simulink model "mobilerobot_DT_SMC"  (R2016b)
settings: Solver=FixedStepAuto  StartTime=0.0  StopTime=20  FixedStep=0.01  RelTol=1e-3
values from neighbouring files (symbols this model uses):
  b = 0.75    [robotprojectvalues.m]
  c = K'    [DTSMC_Gao_TWMR_Position_param.m]    (also in DTSMC_Gao_TWMR_velocity_param.m; robotprojectvalues.m = 0.5)
  c1_pos = c_pos(1)    [robotprojectvalues.m]
  c1_vel = c_vel(1)    [robotprojectvalues.m]
  c2_pos = c_pos(2)    [robotprojectvalues.m]
  c_pos = K_pos'    [robotprojectvalues.m]
  c_vel = K_vel'    [robotprojectvalues.m]
  d = 1    [robotprojectvalues.m]
  dm = 0.1    [robotprojectvalues.m]
  esp = 0.1    [robotprojectvalues.m]
  Gam_tau_pos = [5e-5; 0.01]    [robotprojectvalues.m]
  Gam_tau_vel = [0;1]    [robotprojectvalues.m]
  I_c = 1    [robotprojectvalues.m]
  I_m = 15    [robotprojectvalues.m]
  I_w = 100    [robotprojectvalues.m]
  m1 = a(1)    [robotprojectvalues.m]
  m2 = a(2)    [robotprojectvalues.m]
  m_c = 20    [robotprojectvalues.m]
  m_w = 15    [robotprojectvalues.m]
  mu = 250    [robotprojectvalues.m]
  tau = 0.01    [robotprojectvalues.m]
  x = (1-mu*tau)    (= -1)    [robotprojectvalues.m]
  Xr_c = 5    [robotprojectvalues.m]
  y = dm-esp*tau    (= 0.099)    [robotprojectvalues.m]
  Yr_c = 0    [robotprojectvalues.m]
undefined symbols (not defined in the file or in its folder): fai, Kd, Ki, Kp, theta_dot_L, theta_dot_R
libraries: dspinverses x2, simulink x1
(part 1 of 2)
settings Model: Creator=vasug  LastModifiedBy=HP

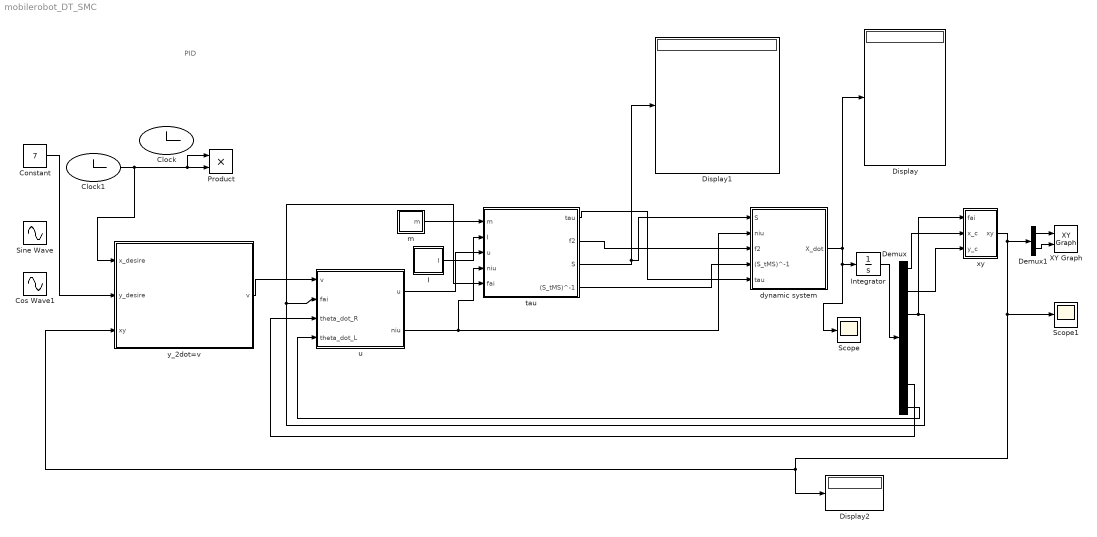
== system mobilerobot_DT_SMC ==
  note: PID
  Clock : Clock
  Clock1 : Clock
  Constant : Constant  Value=7
  Cos Wave1 : Sin  Amplitude=10  Phase=pi/2  SampleTime=0
  Demux : Demux  Outputs=7
  Demux1 : Demux  Outputs=2
  Display : Display
  Display1 : Display
  Display2 : Display
  I : Subsystem
  Integrator : Integrator  InitialCondition=[0; 0; pi/2; 0; 0; 0; 0]
  Product : Product
  Scope : Scope
  Scope1 : Scope
  Sine Wave : Sin  Amplitude=10  SampleTime=0
  XY Graph : simulink/Sinks/XY Graph  xmin=-inf  xmax=inf  ymin=-inf  ymax=inf  st=0.01
  dynamic system : Subsystem
  m : Subsystem
  tau : Subsystem
  "u " : Subsystem
  xy : Subsystem
  y_2dot=v : Subsystem
  wires:
  y_2dot=v/1(v) -> "u "/1(v)
  "u "/1("u ") -> tau/3(u)
  Demux/3 -> xy/1(fai), tau/5(fai), "u "/2(fai)
  tau/4((S_tMS)^-1) -> dynamic system/4((S_tMS)^-1)
  tau/2("f2 ") -> dynamic system/3(f2)
  "u "/2("niu ") -> tau/4(niu), dynamic system/2(niu)
  tau/1(tau) -> dynamic system/5(tau)
  dynamic system/1(X_dot) -> Display/1, Scope/1, Integrator/1
  m/1(m) -> tau/1(m)
  I/1(I) -> tau/2(I)
  xy/1(xy) -> Display2/1, y_2dot=v/3(xy), Scope1/1, Demux1/1
  Demux/1 -> xy/2(x_c)
  Demux/2 -> xy/3(y_c)
  Integrator/1 -> Demux/1
  Demux1/1 -> XY Graph/1
  Demux1/2 -> XY Graph/2
  tau/3("S ") -> Display1/1, dynamic system/1(S)
  Demux/6 -> "u "/3(theta_dot_R)
  Demux/7 -> "u "/4(theta_dot_L)
  Clock1/1 -> y_2dot=v/1(x_desire), Product/1, Product/2
  Constant/1 -> y_2dot=v/2(y_desire)

== system mobilerobot_DT_SMC/I ==
  Constant : Constant  Value=I_c
  Constant1 : Constant  Value=2
  Constant2 : Constant  Value=m_w
  Constant3 : Constant  Value=d
  Constant4 : Constant  Value=b
  Constant5 : Constant  Value=2
  Constant6 : Constant  Value=I_m
  Product : Product
  Product1 : Product  Inputs=3
  Product2 : Product
  Product3 : Product
  Sum : Sum  Inputs=|+++
  Sum1 : Sum  Inputs=|++
  I : Outport
  wires:
  Constant/1 -> Sum/1
  Constant1/1 -> Product1/1
  Constant2/1 -> Product1/2
  Sum1/1 -> Product1/3
  Product1/1 -> Sum/2
  Constant5/1 -> Product/1
  Constant6/1 -> Product/2
  Product/1 -> Sum/3
  Sum/1 -> I/1
  Constant3/1 -> Product2/2, Product2/1
  Product2/1 -> Sum1/1
  Constant4/1 -> Product3/1, Product3/2
  Product3/1 -> Sum1/2

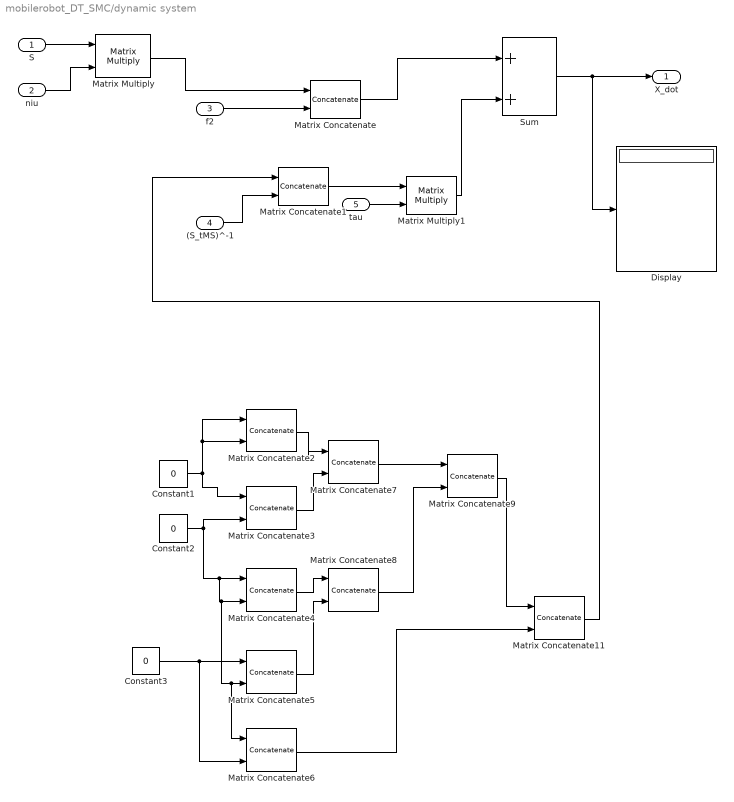
== system mobilerobot_DT_SMC/dynamic system ==
  S : Inport
  niu : Inport  Port=2
  f2 : Inport  Port=3
  (S_tMS)^-1 : Inport  Port=4
  tau : Inport  Port=5
  Constant1 : Constant  Value=0
  Constant2 : Constant  Value=0
  Constant3 : Constant  Value=0
  Display : Display
  Matrix Concatenate{,1,7..9,11} (6 alike) : Concatenate  Mode=Multidimensional array
  Matrix Concatenate{2..6} (5 alike) : Concatenate  Mode=Multidimensional array  ConcatenateDimension=2
  Matrix Multiply : Product  Multiplication=Matrix(*)
  Matrix Multiply1 : Product  Multiplication=Matrix(*)
  Sum : Sum  Inputs=|++
  X_dot : Outport
  wires:
  niu/1 -> Matrix Multiply/2
  S/1 -> Matrix Multiply/1
  Matrix Multiply/1 -> Matrix Concatenate/1
  f2/1 -> Matrix Concatenate/2
  Matrix Concatenate/1 -> Sum/1
  (S_tMS)^-1/1 -> Matrix Concatenate1/2
  Sum/1 -> Display/1, X_dot/1
  Matrix Concatenate1/1 -> Matrix Multiply1/1
  tau/1 -> Matrix Multiply1/2
  Matrix Multiply1/1 -> Sum/2
  Matrix Concatenate6/1 -> Matrix Concatenate11/2
  Matrix Concatenate9/1 -> Matrix Concatenate11/1
  Matrix Concatenate4/1 -> Matrix Concatenate8/1
  Matrix Concatenate5/1 -> Matrix Concatenate8/2
  Matrix Concatenate7/1 -> Matrix Concatenate9/1
  Constant2/1 -> Matrix Concatenate3/2, Matrix Concatenate6/1, Matrix Concatenate5/2, Matrix Concatenate4/2, Matrix Concatenate4/1
  Matrix Concatenate2/1 -> Matrix Concatenate7/1
  Matrix Concatenate3/1 -> Matrix Concatenate7/2
  Matrix Concatenate8/1 -> Matrix Concatenate9/2
  Constant1/1 -> Matrix Concatenate3/1, Matrix Concatenate2/2, Matrix Concatenate2/1
  Matrix Concatenate11/1 -> Matrix Concatenate1/1
  Constant3/1 -> Matrix Concatenate6/2, Matrix Concatenate5/1

== system mobilerobot_DT_SMC/m ==
  Constant : Constant  Value=m_c
  Constant2 : Constant  Value=m_w
  Constant3 : Constant  Value=2
  Product : Product
  Sum : Sum  Inputs=|++
  m : Outport
  wires:
  Constant3/1 -> Product/1
  Constant2/1 -> Product/2
  Product/1 -> Sum/2
  Constant/1 -> Sum/1
  Sum/1 -> m/1

== system mobilerobot_DT_SMC/tau ==
  m : Inport
  I : Inport  Port=2
  u : Inport  Port=3
  niu : Inport  Port=4
  fai : Inport  Port=5
  Derivative : Derivative
  Display : Display
  M : Subsystem
  Matrix Multiply : Product  Inputs=3  Multiplication=Matrix(*)
  Matrix Multiply1 : Product  Multiplication=Matrix(*)
  Product : Product
  S : Subsystem
  "S_transpose " : Subsystem
  Sum : Sum  Inputs=|+-
  f2 : Subsystem
  tau : Outport
  "f2 " : Outport  Port=2
  "S " : Outport  Port=3
  (S_tMS)^-1 : Outport  Port=4
  wires:
  I/1 -> f2/2(I), M/3("I ")
  fai/1 -> Derivative/1, S/1("fai "), f2/3(fai), M/1("fai "), "S_transpose "/1("fai ")
  m/1 -> M/2("m "), f2/1(m)
  "S_transpose "/1(S_t) -> Matrix Multiply/1
  M/1(M) -> Matrix Multiply/2
  S/1(S) -> "S "/1, Matrix Multiply/3
  f2/1(f2) -> Sum/2, "f2 "/1
  u/1 -> Sum/1
  Sum/1 -> Matrix Multiply1/2
  Matrix Multiply/1 -> Matrix Multiply1/1
  Matrix Multiply1/1 -> tau/1
  f2/2((S_tMS)^-1) -> (S_tMS)^-1/1
  Derivative/1 -> Product/2, Product/1
  Product/1 -> Display/1, f2/5((fai_dot)^2)
  niu/1 -> f2/4(niu)

== system mobilerobot_DT_SMC/u  ==
  v : Inport
  fai : Inport  Port=2
  theta_dot_R : Inport  Port=3
  theta_dot_L : Inport  Port=4
  Display4 : Display
  Display8 : Display
  Matrix Multiply : Product  Multiplication=Matrix(*)
  Matrix Multiply1 : Product  Multiplication=Matrix(*)
  Sum : Sum  Inputs=|+-
  faifunction dot : Subsystem
  inverse faifunction : Subsystem
  "niu " : Subsystem
  "u " : Outport
  "niu " : Outport  Port=2
  wires:
  faifunction dot/1(Out1) -> Matrix Multiply/1, Display4/1
  fai/1 -> faifunction dot/1(fai), inverse faifunction/1(fai)
  v/1 -> Sum/1
  inverse faifunction/1(Out1) -> Matrix Multiply1/1, Display8/1
  "niu "/1(Out1) -> Matrix Multiply/2, "niu "/1
  Matrix Multiply/1 -> Sum/2
  Matrix Multiply1/1 -> "u "/1
  Sum/1 -> Matrix Multiply1/2
  theta_dot_L/1 -> "niu "/2(theta_dot_L)
  theta_dot_R/1 -> "niu "/1(theta_dot_R)

== system mobilerobot_DT_SMC/xy ==
  fai : Inport
  x_c : Inport  Port=2
  y_c : Inport  Port=3
  Display : Display
  Matrix Concatenate : Concatenate
  Xr : Subsystem
  Yr : Subsystem
  xy : Outport
  wires:
  Yr/1(Out1) -> Matrix Concatenate/2
  Matrix Concatenate/1 -> Display/1, xy/1
  Xr/1(Out1) -> Matrix Concatenate/1
  fai/1 -> Xr/1(fai), Yr/1("fai ")
  x_c/1 -> Xr/2(Xc)
  y_c/1 -> Yr/2("Yc ")

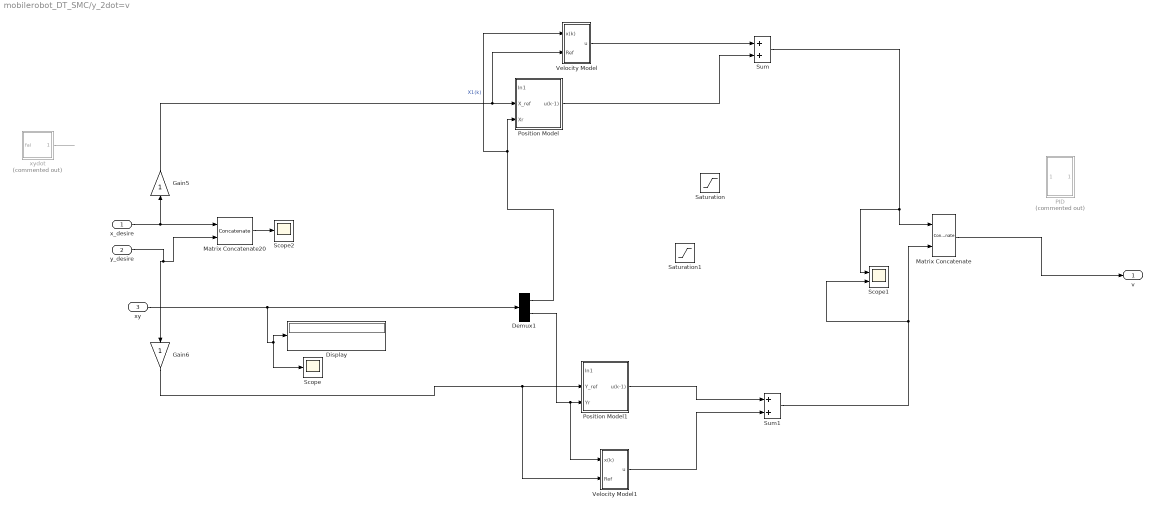
== system mobilerobot_DT_SMC/y_2dot=v ==
  x_desire : Inport
  y_desire : Inport  Port=2
  xy : Inport  Port=3
  Demux1 : Demux  Outputs=2
  Display : Display
  Gain5 : Gain
  Gain6 : Gain
  Matrix Concatenate : Concatenate  Mode=Multidimensional array
  Matrix Concatenate20 : Concatenate  Mode=Multidimensional array
  PID : Subsystem  Commented=on
  Position Model : Subsystem
  Position Model1 : Subsystem
  Saturation : Saturate  UpperLimit=50  LowerLimit=-50  LinearizeAsGain=off
  Saturation1 : Saturate  UpperLimit=50  LowerLimit=-50  LinearizeAsGain=off
  Scope : Scope
  Scope1 : Scope  NumInputPorts=2
  Scope2 : Scope
  Sum : Sum
  Sum1 : Sum
  Velocity Model : Subsystem
  Velocity Model1 : Subsystem
  xydot : Subsystem  Commented=on
  v : Outport
  wires:
  xydot/1(Out1) -> ?
  xy/1 -> Demux1/1, Scope/1, Display/1
  Matrix Concatenate/1 -> v/1
  x_desire/1 -> Matrix Concatenate20/1, Gain5/1
  y_desire/1 -> Matrix Concatenate20/2, Gain6/1
  Matrix Concatenate20/1 -> Scope2/1
  Gain5/1 -> Velocity Model/2(Ref), Position Model/2(X_ref)
  Demux1/1 -> Velocity Model/1(x(k)), Position Model/3(Xr)  "X1(k)"
  Velocity Model/1(u) -> Sum/1
  Position Model/1(u(k-1)) -> Sum/2
  Sum/1 -> Scope1/1, Matrix Concatenate/1
  Gain6/1 -> Velocity Model1/2(Ref), Position Model1/2(Y_ref)
  Demux1/2 -> Velocity Model1/1(x(k)), Position Model1/3(Yr)
  Velocity Model1/1(u) -> Sum1/2
  Position Model1/1(u(k-1)) -> Sum1/1
  Sum1/1 -> Scope1/2, Matrix Concatenate/2

== system mobilerobot_DT_SMC/tau/M ==
  "fai " : Inport
  "m " : Inport  Port=2
  "I " : Inport  Port=3
  Constant : Constant  Value=I_w
  Constant1 : Constant  Value=0
  Constant3 : Constant  Value=0
  Constant5 : Constant  Value=0
  Matrix Concatenate{,1..4} (5 alike) : Concatenate  NumInputs=5  Mode=Multidimensional array  ConcatenateDimension=2
  Matrix Concatenate7 : Concatenate  NumInputs=5  Mode=Multidimensional array
  Subsystem : Subsystem
  Subsystem1 : Subsystem
  M : Outport
  wires:
  "m "/1 -> Matrix Concatenate1/2, Matrix Concatenate/1
  Constant5/1 -> Matrix Concatenate/2
  "fai "/1 -> Subsystem1/1(fai), Subsystem/1("fai ")
  Subsystem/1(Out1) -> Matrix Concatenate2/1, Matrix Concatenate/3
  Constant1/1 -> Matrix Concatenate/4
  Constant3/1 -> Matrix Concatenate3/2, Matrix Concatenate4/4, Matrix Concatenate4/3, Matrix Concatenate4/2, Matrix Concatenate4/1, Matrix Concatenate3/5, Matrix Concatenate3/3, Matrix Concatenate3/1, Matrix Concatenate2/5, Matrix Concatenate2/4, Matrix Concatenate1/5, Matrix Concatenate1/4, Matrix Concatenate1/1, Matrix Concatenate/5
  Subsystem1/1(Out1) -> Matrix Concatenate2/2, Matrix Concatenate1/3
  "I "/1 -> Matrix Concatenate2/3
  Constant/1 -> Matrix Concatenate4/5, Matrix Concatenate3/4
  Matrix Concatenate/1 -> Matrix Concatenate7/1
  Matrix Concatenate1/1 -> Matrix Concatenate7/2
  Matrix Concatenate2/1 -> Matrix Concatenate7/3
  Matrix Concatenate3/1 -> Matrix Concatenate7/4
  Matrix Concatenate4/1 -> Matrix Concatenate7/5
  Matrix Concatenate7/1 -> M/1

== system mobilerobot_DT_SMC/tau/S ==
  "fai " : Inport
  Constant19 : Constant  Value=c
  Constant20 : Constant  Value=-c
  Constant21 : Constant
  Constant22 : Constant  Value=0
  Constant23 : Constant  Value=0
  Constant24 : Constant
  Matrix Concatenate{1,3..6} (5 alike) : Concatenate  Mode=Multidimensional array  ConcatenateDimension=2
  Matrix Concatenate{7..9,11} (4 alike) : Concatenate  Mode=Multidimensional array
  Subsystem : Subsystem
  Subsystem1 : Subsystem
  Subsystem2 : Subsystem
  Subsystem3 : Subsystem
  S : Outport
  wires:
  Constant19/1 -> Matrix Concatenate4/1
  Constant23/1 -> Matrix Concatenate5/2
  Constant21/1 -> Matrix Concatenate5/1
  Matrix Concatenate6/1 -> Matrix Concatenate11/2
  Subsystem3/1(Out1) -> Matrix Concatenate1/1
  Subsystem2/1(Out1) -> Matrix Concatenate1/2
  Matrix Concatenate9/1 -> Matrix Concatenate11/1
  Subsystem1/1(Out1) -> Matrix Concatenate3/1
  Matrix Concatenate4/1 -> Matrix Concatenate8/1
  Constant24/1 -> Matrix Concatenate6/2
  Matrix Concatenate5/1 -> Matrix Concatenate8/2
  Matrix Concatenate7/1 -> Matrix Concatenate9/1
  Subsystem/1(Out1) -> Matrix Concatenate3/2
  Constant20/1 -> Matrix Concatenate4/2
  Matrix Concatenate1/1 -> Matrix Concatenate7/1
  Matrix Concatenate3/1 -> Matrix Concatenate7/2
  Matrix Concatenate8/1 -> Matrix Concatenate9/2
  Matrix Concatenate11/1 -> S/1
  Constant22/1 -> Matrix Concatenate6/1
  "fai "/1 -> Subsystem/1("fai "), Subsystem1/1("fai "), Subsystem2/1("fai "), Subsystem3/1("fai ")

== system mobilerobot_DT_SMC/tau/S_transpose  ==
  "fai " : Inport
  Constant19 : Constant  Value=c
  Constant20 : Constant  Value=-c
  Constant21 : Constant
  Constant22 : Constant  Value=0
  Constant23 : Constant  Value=0
  Constant24 : Constant
  Matrix Concatenate{1,3..6} (5 alike) : Concatenate  Mode=Multidimensional array
  Matrix Concatenate{7..9,11} (4 alike) : Concatenate  Mode=Multidimensional array  ConcatenateDimension=2
  Subsystem : Subsystem
  Subsystem1 : Subsystem
  Subsystem2 : Subsystem
  Subsystem3 : Subsystem
  S_t : Outport
  wires:
  Subsystem/1(Out1) -> Matrix Concatenate3/2
  Constant20/1 -> Matrix Concatenate4/2
  Matrix Concatenate1/1 -> Matrix Concatenate7/1
  Subsystem3/1(Out1) -> Matrix Concatenate1/1
  "fai "/1 -> Subsystem/1("fai "), Subsystem1/1("fai "), Subsystem2/1("fai "), Subsystem3/1("fai ")
  Matrix Concatenate3/1 -> Matrix Concatenate7/2
  Constant19/1 -> Matrix Concatenate4/1
  Matrix Concatenate7/1 -> Matrix Concatenate9/1
  Constant24/1 -> Matrix Concatenate6/2
  Constant22/1 -> Matrix Concatenate6/1
  Matrix Concatenate9/1 -> Matrix Concatenate11/1
  Matrix Concatenate5/1 -> Matrix Concatenate8/2
  Constant21/1 -> Matrix Concatenate5/1
  Matrix Concatenate6/1 -> Matrix Concatenate11/2
  Subsystem1/1(Out1) -> Matrix Concatenate3/1
  Matrix Concatenate8/1 -> Matrix Concatenate9/2
  Subsystem2/1(Out1) -> Matrix Concatenate1/2
  Matrix Concatenate4/1 -> Matrix Concatenate8/1
  Matrix Concatenate11/1 -> S_t/1
  Constant23/1 -> Matrix Concatenate5/2

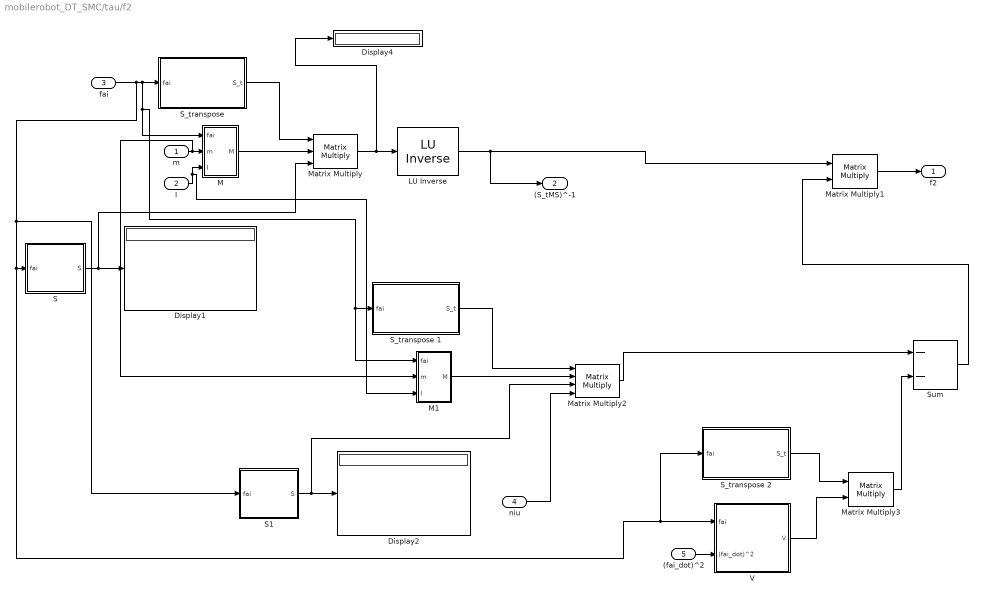
== system mobilerobot_DT_SMC/tau/f2 ==
  m : Inport
  I : Inport  Port=2
  fai : Inport  Port=3
  niu : Inport  Port=4
  (fai_dot)^2 : Inport  Port=5
  " LU Inverse" : dspinverses/ LU Inverse
  Display1 : Display
  Display2 : Display
  Display4 : Display
  M : Subsystem
  M1 : Subsystem
  Matrix Multiply : Product  Inputs=3  Multiplication=Matrix(*)
  Matrix Multiply1 : Product  Multiplication=Matrix(*)
  Matrix Multiply2 : Product  Inputs=4  Multiplication=Matrix(*)
  Matrix Multiply3 : Product  Multiplication=Matrix(*)
  S : Subsystem
  S1 : Subsystem
  "S_transpose " : Subsystem
  S_transpose 1 : Subsystem
  S_transpose 2 : Subsystem
  Sum : Sum  Inputs=--
  V : Subsystem
  f2 : Outport
  (S_tMS)^-1 : Outport  Port=2
  wires:
  S/1(S) -> Matrix Multiply/3, Display1/1
  "S_transpose "/1(S_t) -> Matrix Multiply/1
  M/1(M) -> Matrix Multiply/2
  Matrix Multiply/1 -> Display4/1, " LU Inverse"/1
  I/1 -> M1/3("I "), M/3("I ")
  S1/1(S) -> Matrix Multiply2/3, Display2/1
  S_transpose 1/1(S_t) -> Matrix Multiply2/1
  M1/1(M) -> Matrix Multiply2/2
  m/1 -> M1/2("m "), M/2("m ")
  niu/1 -> Matrix Multiply2/4
  fai/1 -> S1/1("fai "), S_transpose 2/1("fai "), V/1(fai), S/1("fai "), M1/1("fai "), S_transpose 1/1("fai "), M/1("fai "), "S_transpose "/1("fai ")
  (fai_dot)^2/1 -> V/2((fai_dot)^2)
  S_transpose 2/1(S_t) -> Matrix Multiply3/1
  V/1(V) -> Matrix Multiply3/2
  Matrix Multiply3/1 -> Sum/2
  Matrix Multiply2/1 -> Sum/1
  " LU Inverse"/1 -> (S_tMS)^-1/1, Matrix Multiply1/1
  Sum/1 -> Matrix Multiply1/2
  Matrix Multiply1/1 -> f2/1

== system mobilerobot_DT_SMC/u /faifunction dot ==
  fai : Inport
  Matrix Concatenate14 : Concatenate  Mode=Multidimensional array  ConcatenateDimension=2
  Matrix Concatenate15 : Concatenate  Mode=Multidimensional array  ConcatenateDimension=2
  Matrix Concatenate16 : Concatenate  Mode=Multidimensional array
  Subsystem10 : Subsystem
  Subsystem11 : Subsystem
  Subsystem12 : Subsystem
  Subsystem13 : Subsystem
  Out1 : Outport
  wires:
  Matrix Concatenate15/1 -> Matrix Concatenate16/2
  Subsystem10/1(Out1) -> Matrix Concatenate14/1
  Subsystem11/1(Out1) -> Matrix Concatenate14/2
  Subsystem13/1(Out1) -> Matrix Concatenate15/2
  Matrix Concatenate14/1 -> Matrix Concatenate16/1
  Matrix Concatenate16/1 -> Out1/1
  Subsystem12/1(Out1) -> Matrix Concatenate15/1
  fai/1 -> Subsystem13/1(fai), Subsystem12/1(fai), Subsystem11/1(fai), Subsystem10/1(fai)

== system mobilerobot_DT_SMC/u /inverse faifunction ==
  fai : Inport
  " LU Inverse" : dspinverses/ LU Inverse
  Matrix Concatenate10 : Concatenate  Mode=Multidimensional array  ConcatenateDimension=2
  Matrix Concatenate12 : Concatenate  Mode=Multidimensional array
  Matrix Concatenate2 : Concatenate  Mode=Multidimensional array  ConcatenateDimension=2
  Subsystem4 : Subsystem
  Subsystem5 : Subsystem
  Subsystem6 : Subsystem
  Subsystem7 : Subsystem
  Out1 : Outport
  wires:
  Subsystem4/1(Out1) -> Matrix Concatenate2/1
  Subsystem5/1(Out1) -> Matrix Concatenate2/2
  Subsystem6/1(Out1) -> Matrix Concatenate10/1
  Matrix Concatenate10/1 -> Matrix Concatenate12/2
  Subsystem7/1(Out1) -> Matrix Concatenate10/2
  Matrix Concatenate2/1 -> Matrix Concatenate12/1
  Matrix Concatenate12/1 -> " LU Inverse"/1
  " LU Inverse"/1 -> Out1/1
  fai/1 -> Subsystem7/1("fai "), Subsystem6/1("fai "), Subsystem5/1("fai "), Subsystem4/1("fai ")

== system mobilerobot_DT_SMC/u /niu  ==
  theta_dot_R : Inport
  theta_dot_L : Inport  Port=2
  Matrix Concatenate23 : Concatenate  Mode=Multidimensional array
  Out1 : Outport
  wires:
  theta_dot_R/1 -> Matrix Concatenate23/1
  theta_dot_L/1 -> Matrix Concatenate23/2
  Matrix Concatenate23/1 -> Out1/1

== system mobilerobot_DT_SMC/xy/Xr ==
  fai : Inport
  Xc : Inport  Port=2
  Constant1 : Constant  Value=Yr_c
  Constant2 : Constant  Value=Xr_c
  Product : Product
  Product1 : Product
  Sum : Sum  Inputs=|++
  Sum1 : Sum  Inputs=|+-
  Trigonometric Function : Trigonometry  Operator=cos
  Trigonometric Function1 : Trigonometry
  Out1 : Outport
  wires:
  Trigonometric Function/1 -> Product/1
  Constant2/1 -> Product/2
  Xc/1 -> Sum/1
  Product/1 -> Sum/2
  fai/1 -> Trigonometric Function1/1, Trigonometric Function/1
  Constant1/1 -> Product1/1
  Trigonometric Function1/1 -> Product1/2
  Sum/1 -> Sum1/1
  Product1/1 -> Sum1/2
  Sum1/1 -> Out1/1

== system mobilerobot_DT_SMC/xy/Yr ==
  "fai " : Inport
  "Yc " : Inport  Port=2
  Constant1 : Constant  Value=Yr_c
  Constant5 : Constant  Value=Xr_c
  Product1 : Product
  Product2 : Product
  Sum1 : Sum  Inputs=|++
  Sum2 : Sum  Inputs=|++
  Trigonometric Function1 : Trigonometry
  Trigonometric Function2 : Trigonometry  Operator=cos
  Out1 : Outport
  wires:
  "fai "/1 -> Trigonometric Function2/1, Trigonometric Function1/1
  Product1/1 -> Sum1/2
  Trigonometric Function1/1 -> Product1/1
  Constant5/1 -> Product1/2
  "Yc "/1 -> Sum1/1
  Constant1/1 -> Product2/1
  Trigonometric Function2/1 -> Product2/2
  Sum1/1 -> Sum2/1
  Product2/1 -> Sum2/2
  Sum2/1 -> Out1/1

== system mobilerobot_DT_SMC/y_2dot=v/PID ==
  In1 : Inport
  Constant1 : Constant  Value=0
  Constant3 : Constant  Value=Kd
  Constant4 : Constant  Value=Kp
  Derivative : Derivative
  Gain : Gain  Gain=Ki
  Integrator : Integrator
  Product : Product
  Product1 : Product
  Sum : Sum  Inputs=++++
  Out1 : Outport
  wires:
  Sum/1 -> Out1/1
  In1/1 -> Product1/2, Integrator/1, Derivative/1
  Derivative/1 -> Product/2
  Constant4/1 -> Product1/1
  Product/1 -> Sum/3
  Integrator/1 -> Gain/1
  Constant3/1 -> Product/1
  Gain/1 -> Sum/2
  Constant1/1 -> Sum/4
  Product1/1 -> Sum/1

== system mobilerobot_DT_SMC/y_2dot=v/Position Model ==
  note: Feedback
  In1 : Inport
  X_ref : Inport  Port=2
  Xr : Inport  Port=3
  Add4 : Sum
  Add5 : Sum
  Add8 : Sum  Inputs=+-
  Gain1 : Gain  Gain=-c1_pos*x
  Gain4 : Gain  Gain=c1_pos
  Subsystem : Subsystem
  Unit Delay : UnitDelay  SampleTime=0.01
  Unit Delay3 : UnitDelay  SampleTime=0.1
  Unit Delay4 : UnitDelay  Commented=on  SampleTime=0.01
  ct_Gamt_inv : Gain  Gain=(c_pos'*Gam_tau_pos)^(-1)  Multiplication=Matrix(K*u)
  u(k-1) : Outport
  wires:
  In1/1 -> Add5/1
  Add8/1 -> ct_Gamt_inv/1  "(k-1)"
  Unit Delay3/1 -> Gain1/1  "x1(k-1)"
  Subsystem/1(Out1) -> Add8/2
  Gain4/1 -> Add4/2
  Add5/1 -> Add8/1  "x2(k+1)"
  Unit Delay/1 -> Subsystem/2(X2(k-2))  "X2(k-1)"
  Add4/1 -> Add5/2  "X11r"
  Gain1/1 -> Add4/1
  X_ref/1 -> Unit Delay3/1, Gain4/1
  Xr/1 -> Unit Delay/1, Subsystem/1(X1(k-1))  "X1(k-1)"
  ct_Gamt_inv/1 -> u(k-1)/1

== system mobilerobot_DT_SMC/y_2dot=v/Position Model1 ==
  note: Feedback
  In1 : Inport
  Y_ref : Inport  Port=2
  Yr : Inport  Port=3
  Add4 : Sum
  Add5 : Sum
  Add8 : Sum  Inputs=+-
  Gain1 : Gain  Gain=-c1_pos*x
  Gain4 : Gain  Gain=c1_pos
  Subsystem : Subsystem
  Unit Delay : UnitDelay  SampleTime=0.01
  Unit Delay3 : UnitDelay  SampleTime=0.1
  Unit Delay4 : UnitDelay  Commented=on  SampleTime=0.01
  ct_Gamt_inv : Gain  Gain=(c_pos'*Gam_tau_pos)^(-1)  Multiplication=Matrix(K*u)
  u(k-1) : Outport
  wires:
  In1/1 -> Add5/1
  Add8/1 -> ct_Gamt_inv/1  "(k-1)"
  Unit Delay3/1 -> Gain1/1  "x1(k-1)"
  Subsystem/1(Out1) -> Add8/2
  Gain4/1 -> Add4/2
  Add5/1 -> Add8/1  "x2(k+1)"
  Unit Delay/1 -> Subsystem/2(X2(k-1))  "X2(k-1)"
  Add4/1 -> Add5/2  "X11r"
  Gain1/1 -> Add4/1
  Y_ref/1 -> Unit Delay3/1, Gain4/1
  Yr/1 -> Unit Delay/1, Subsystem/1(X1(k-1))  "X1(k-1)"
  ct_Gamt_inv/1 -> u(k-1)/1

== system mobilerobot_DT_SMC/y_2dot=v/Velocity Model ==
  x(k) : Inport
  Ref : Inport  Port=2
  Add2 : Sum
  Add3 : Sum  Inputs=+-
  Gain2 : Gain  Gain=c1_vel
  Gain3 : Gain  Gain=-c1_vel*(1-(mu*tau))
  Gain9 : Gain  Gain=(c_vel'*Gam_tau_vel)^-1
  Saturation1 : Saturate  UpperLimit=3.5  LowerLimit=-3.5
  Subsystem1 : Subsystem
  Unit Delay1 : UnitDelay  SampleTime=0.01
  Unit Delay2 : UnitDelay  SampleTime=0.01
  Unit Delay5 : UnitDelay  SampleTime=0.01
  u : Outport
  wires:
  Unit Delay5/1 -> Saturation1/1  "u(k-2)"
  Unit Delay2/1 -> Gain3/1  "xr(k-1)"
  Gain2/1 -> Add2/1
  x(k)/1 -> Subsystem1/1(X(k-1))  "x(k-1)"
  Gain3/1 -> Add2/2
  Add2/1 -> Add3/1  "x(k))"
  Ref/1 -> Gain2/1, Unit Delay2/1
  Saturation1/1 -> u/1, Subsystem1/2(u(k-2))
  Subsystem1/1(Out1) -> Add3/2
  Add3/1 -> Gain9/1
  Gain9/1 -> Unit Delay5/1  "u(k-1)"

== system mobilerobot_DT_SMC/y_2dot=v/Velocity Model1 ==
  x(k) : Inport
  Ref : Inport  Port=2
  Add2 : Sum
  Add3 : Sum  Inputs=+-
  Gain2 : Gain  Gain=c1_vel
  Gain3 : Gain  Gain=-c1_vel*(1-(mu*tau))
  Gain9 : Gain  Gain=(c_vel'*Gam_tau_vel)^-1
  Saturation1 : Saturate  UpperLimit=3.5  LowerLimit=-3.5
  Subsystem1 : Subsystem
  Unit Delay1 : UnitDelay  Commented=on  SampleTime=0.01
  Unit Delay2 : UnitDelay  SampleTime=0.01
  Unit Delay5 : UnitDelay  SampleTime=0.01
  u : Outport
  wires:
  Unit Delay5/1 -> Saturation1/1  "u(k-2)"
  Unit Delay2/1 -> Gain3/1  "xr(k-1)"
  Gain2/1 -> Add2/1
  x(k)/1 -> Subsystem1/1(X(k-1))  "x(k-1)"
  Gain3/1 -> Add2/2
  Add2/1 -> Add3/1  "x(k))"
  Ref/1 -> Gain2/1, Unit Delay2/1
  Saturation1/1 -> u/1, Subsystem1/2(u(k-2))
  Subsystem1/1(Out1) -> Add3/2
  Add3/1 -> Gain9/1
  Gain9/1 -> Unit Delay5/1  "u(k-1)"

== system mobilerobot_DT_SMC/y_2dot=v/xydot ==
  fai : Inport
  Constant1 : Constant  Value=theta_dot_R
  Constant2 : Constant  Value=theta_dot_L
  Matrix Concatenate10 : Concatenate  Mode=Multidimensional array  ConcatenateDimension=2
  Matrix Concatenate12 : Concatenate  Mode=Multidimensional array
  Matrix Concatenate13 : Concatenate  Mode=Multidimensional array
  Matrix Concatenate2 : Concatenate  Mode=Multidimensional array  ConcatenateDimension=2
  Matrix Multiply : Product  Multiplication=Matrix(*)
  Subsystem4 : Subsystem
  Subsystem5 : Subsystem
  Subsystem6 : Subsystem
  Subsystem7 : Subsystem
  Out1 : Outport
  wires:
  Matrix Concatenate12/1 -> Matrix Multiply/1
  Constant2/1 -> Matrix Concatenate13/2
  Constant1/1 -> Matrix Concatenate13/1
  Matrix Multiply/1 -> Out1/1
  Matrix Concatenate13/1 -> Matrix Multiply/2
  Subsystem4/1(Out1) -> Matrix Concatenate2/1
  Subsystem5/1(Out1) -> Matrix Concatenate2/2
  Subsystem6/1(Out1) -> Matrix Concatenate10/1
  Matrix Concatenate10/1 -> Matrix Concatenate12/2
  Subsystem7/1(Out1) -> Matrix Concatenate10/2
  Matrix Concatenate2/1 -> Matrix Concatenate12/1
  fai/1 -> Subsystem7/1("fai "), Subsystem6/1("fai "), Subsystem5/1("fai "), Subsystem4/1("fai ")

== system mobilerobot_DT_SMC/tau/M/Subsystem ==
  "fai " : Inport
  Constant : Constant  Value=-m_c
  Constant1 : Constant  Value=d
  Product : Product
  Product1 : Product
  Trigonometric Function : Trigonometry
  Out1 : Outport
  wires:
  Trigonometric Function/1 -> Product/2
  "fai "/1 -> Trigonometric Function/1
  Constant/1 -> Product1/1
  Constant1/1 -> Product/1
  Product1/1 -> Out1/1
  Product/1 -> Product1/2

== system mobilerobot_DT_SMC/tau/M/Subsystem1 ==
  fai : Inport
  Constant3 : Constant  Value=m_c
  Constant4 : Constant  Value=d
  Product2 : Product
  Product3 : Product
  Trigonometric Function1 : Trigonometry
  Out1 : Outport
  wires:
  Trigonometric Function1/1 -> Product2/2
  Constant4/1 -> Product2/1
  fai/1 -> Trigonometric Function1/1
  Product2/1 -> Product3/2
  Constant3/1 -> Product3/1
  Product3/1 -> Out1/1

== system mobilerobot_DT_SMC/tau/S/Subsystem ==
  "fai " : Inport
  Constant16 : Constant  Value=c
  Constant17 : Constant  Value=b
  Constant18 : Constant  Value=d
  Product11 : Product
  Product12 : Product
  Product13 : Product
  Sum5 : Sum  Inputs=|+-
  Trigonometric Function8 : Trigonometry
  Trigonometric Function9 : Trigonometry  Operator=cos
  Out1 : Outport
  wires:
  Constant17/1 -> Product13/1
  Product12/1 -> Sum5/2
  Product13/1 -> Sum5/1
  Constant16/1 -> Product11/1
  Product11/1 -> Out1/1
  Constant18/1 -> Product12/1
  Sum5/1 -> Product11/2
  Trigonometric Function8/1 -> Product13/2
  Trigonometric Function9/1 -> Product12/2
  "fai "/1 -> Trigonometric Function9/1, Trigonometric Function8/1

== system mobilerobot_DT_SMC/tau/S/Subsystem1 ==
  "fai " : Inport
  Constant13 : Constant  Value=c
  Constant14 : Constant  Value=b
  Constant15 : Constant  Value=d
  Product10 : Product
  Product8 : Product
  Product9 : Product
  Sum4 : Sum  Inputs=|++
  Trigonometric Function6 : Trigonometry
  Trigonometric Function7 : Trigonometry  Operator=cos
  Out1 : Outport
  wires:
  Product10/1 -> Out1/1
  Sum4/1 -> Product10/2
  Product9/1 -> Sum4/1
  Trigonometric Function6/1 -> Product9/2
  Product8/1 -> Sum4/2
  Constant14/1 -> Product9/1
  Constant15/1 -> Product8/1
  Trigonometric Function7/1 -> Product8/2
  Constant13/1 -> Product10/1
  "fai "/1 -> Trigonometric Function7/1, Trigonometric Function6/1

== system mobilerobot_DT_SMC/tau/S/Subsystem2 ==
  "fai " : Inport
  Constant10 : Constant  Value=c
  Constant11 : Constant  Value=b
  Constant12 : Constant  Value=d
  Product5 : Product
  Product6 : Product
  Product7 : Product
  Sum3 : Sum  Inputs=|++
  Trigonometric Function4 : Trigonometry  Operator=cos
  Trigonometric Function5 : Trigonometry
  Out1 : Outport
  wires:
  Constant11/1 -> Product6/1
  Trigonometric Function4/1 -> Product6/2
  Constant12/1 -> Product5/1
  Trigonometric Function5/1 -> Product5/2
  Product6/1 -> Sum3/1
  Product5/1 -> Sum3/2
  Constant10/1 -> Product7/1
  Sum3/1 -> Product7/2
  Product7/1 -> Out1/1
  "fai "/1 -> Trigonometric Function5/1, Trigonometric Function4/1

== system mobilerobot_DT_SMC/tau/S/Subsystem3 ==
  "fai " : Inport
  Constant6 : Constant  Value=c
  Constant7 : Constant  Value=b
  Constant8 : Constant  Value=d
  Product2 : Product
  Product3 : Product
  Product4 : Product
  Sum2 : Sum  Inputs=|+-
  Trigonometric Function2 : Trigonometry  Operator=cos
  Trigonometric Function3 : Trigonometry
  Out1 : Outport
  wires:
  Sum2/1 -> Product4/2
  Trigonometric Function3/1 -> Product2/2
  Constant8/1 -> Product2/1
  Trigonometric Function2/1 -> Product3/2
  Constant7/1 -> Product3/1
  Product3/1 -> Sum2/1
  Constant6/1 -> Product4/1
  Product2/1 -> Sum2/2
  Product4/1 -> Out1/1
  "fai "/1 -> Trigonometric Function3/1, Trigonometric Function2/1

== system mobilerobot_DT_SMC/tau/S_transpose /Subsystem ==
  "fai " : Inport
  Constant16 : Constant  Value=c
  Constant17 : Constant  Value=b
  Constant18 : Constant
  Product11 : Product
  Product12 : Product
  Product13 : Product
  Sum5 : Sum  Inputs=|+-
  Trigonometric Function8 : Trigonometry
  Trigonometric Function9 : Trigonometry  Operator=cos
  Out1 : Outport
  wires:
  Constant17/1 -> Product13/1
  Product12/1 -> Sum5/2
  Product13/1 -> Sum5/1
  Constant16/1 -> Product11/1
  Product11/1 -> Out1/1
  Constant18/1 -> Product12/1
  Sum5/1 -> Product11/2
  Trigonometric Function8/1 -> Product13/2
  Trigonometric Function9/1 -> Product12/2
  "fai "/1 -> Trigonometric Function9/1, Trigonometric Function8/1

== system mobilerobot_DT_SMC/tau/S_transpose /Subsystem1 ==
  "fai " : Inport
  Constant13 : Constant  Value=c
  Constant14 : Constant  Value=b
  Constant15 : Constant
  Product10 : Product
  Product8 : Product
  Product9 : Product
  Sum4 : Sum  Inputs=|++
  Trigonometric Function6 : Trigonometry
  Trigonometric Function7 : Trigonometry  Operator=cos
  Out1 : Outport
  wires:
  Product10/1 -> Out1/1
  Sum4/1 -> Product10/2
  Product9/1 -> Sum4/1
  Trigonometric Function6/1 -> Product9/2
  Product8/1 -> Sum4/2
  Constant14/1 -> Product9/1
  Constant15/1 -> Product8/1
  Trigonometric Function7/1 -> Product8/2
  Constant13/1 -> Product10/1
  "fai "/1 -> Trigonometric Function7/1, Trigonometric Function6/1

== system mobilerobot_DT_SMC/tau/S_transpose /Subsystem2 ==
  "fai " : Inport
  Constant10 : Constant  Value=c
  Constant11 : Constant  Value=b
  Constant12 : Constant
  Product5 : Product
  Product6 : Product
  Product7 : Product
  Sum3 : Sum  Inputs=|++
  Trigonometric Function4 : Trigonometry  Operator=cos
  Trigonometric Function5 : Trigonometry
  Out1 : Outport
  wires:
  Constant11/1 -> Product6/1
  Trigonometric Function4/1 -> Product6/2
  Constant12/1 -> Product5/1
  Trigonometric Function5/1 -> Product5/2
  Product6/1 -> Sum3/1
  Product5/1 -> Sum3/2
  Constant10/1 -> Product7/1
  Sum3/1 -> Product7/2
  Product7/1 -> Out1/1
  "fai "/1 -> Trigonometric Function5/1, Trigonometric Function4/1

== system mobilerobot_DT_SMC/tau/S_transpose /Subsystem3 ==
  "fai " : Inport
  Constant6 : Constant  Value=c
  Constant7 : Constant  Value=b
  Constant8 : Constant
  Product2 : Product
  Product3 : Product
  Product4 : Product
  Sum2 : Sum  Inputs=|+-
  Trigonometric Function2 : Trigonometry  Operator=cos
  Trigonometric Function3 : Trigonometry
  Out1 : Outport
  wires:
  Sum2/1 -> Product4/2
  Trigonometric Function3/1 -> Product2/2
  Constant8/1 -> Product2/1
  Trigonometric Function2/1 -> Product3/2
  Constant7/1 -> Product3/1
  Product3/1 -> Sum2/1
  Constant6/1 -> Product4/1
  Product2/1 -> Sum2/2
  Product4/1 -> Out1/1
  "fai "/1 -> Trigonometric Function3/1, Trigonometric Function2/1

== system mobilerobot_DT_SMC/tau/f2/M ==
  "fai " : Inport
  "m " : Inport  Port=2
  "I " : Inport  Port=3
  Constant : Constant  Value=I_w
  Constant1 : Constant  Value=0
  Constant3 : Constant  Value=0
  Constant5 : Constant  Value=0
  Matrix Concatenate{,1..4} (5 alike) : Concatenate  NumInputs=5  Mode=Multidimensional array  ConcatenateDimension=2
  Matrix Concatenate7 : Concatenate  NumInputs=5  Mode=Multidimensional array
  Subsystem : Subsystem
  Subsystem1 : Subsystem
  M : Outport
  wires:
  "m "/1 -> Matrix Concatenate1/2, Matrix Concatenate/1
  Constant5/1 -> Matrix Concatenate/2
  "fai "/1 -> Subsystem1/1(fai), Subsystem/1("fai ")
  Subsystem/1(Out1) -> Matrix Concatenate2/1, Matrix Concatenate/3
  Constant1/1 -> Matrix Concatenate/4
  Constant3/1 -> Matrix Concatenate3/2, Matrix Concatenate4/4, Matrix Concatenate4/3, Matrix Concatenate4/2, Matrix Concatenate4/1, Matrix Concatenate3/5, Matrix Concatenate3/3, Matrix Concatenate3/1, Matrix Concatenate2/5, Matrix Concatenate2/4, Matrix Concatenate1/5, Matrix Concatenate1/4, Matrix Concatenate1/1, Matrix Concatenate/5
  Subsystem1/1(Out1) -> Matrix Concatenate2/2, Matrix Concatenate1/3
  "I "/1 -> Matrix Concatenate2/3
  Constant/1 -> Matrix Concatenate4/5, Matrix Concatenate3/4
  Matrix Concatenate/1 -> Matrix Concatenate7/1
  Matrix Concatenate1/1 -> Matrix Concatenate7/2
  Matrix Concatenate2/1 -> Matrix Concatenate7/3
  Matrix Concatenate3/1 -> Matrix Concatenate7/4
  Matrix Concatenate4/1 -> Matrix Concatenate7/5
  Matrix Concatenate7/1 -> M/1

== system mobilerobot_DT_SMC/tau/f2/M1 ==
  "fai " : Inport
  "m " : Inport  Port=2
  "I " : Inport  Port=3
  Constant : Constant  Value=I_w
  Constant1 : Constant  Value=0
  Constant3 : Constant  Value=0
  Constant5 : Constant  Value=0
  Matrix Concatenate{,1..4} (5 alike) : Concatenate  NumInputs=5  Mode=Multidimensional array  ConcatenateDimension=2
  Matrix Concatenate7 : Concatenate  NumInputs=5  Mode=Multidimensional array
  Subsystem : Subsystem
  Subsystem1 : Subsystem
  M : Outport
  wires:
  "m "/1 -> Matrix Concatenate1/2, Matrix Concatenate/1
  Constant5/1 -> Matrix Concatenate/2
  "fai "/1 -> Subsystem1/1(fai), Subsystem/1("fai ")
  Subsystem/1(Out1) -> Matrix Concatenate2/1, Matrix Concatenate/3
  Constant1/1 -> Matrix Concatenate/4
  Constant3/1 -> Matrix Concatenate3/2, Matrix Concatenate4/4, Matrix Concatenate4/3, Matrix Concatenate4/2, Matrix Concatenate4/1, Matrix Concatenate3/5, Matrix Concatenate3/3, Matrix Concatenate3/1, Matrix Concatenate2/5, Matrix Concatenate2/4, Matrix Concatenate1/5, Matrix Concatenate1/4, Matrix Concatenate1/1, Matrix Concatenate/5
  Subsystem1/1(Out1) -> Matrix Concatenate2/2, Matrix Concatenate1/3
  "I "/1 -> Matrix Concatenate2/3
  Constant/1 -> Matrix Concatenate4/5, Matrix Concatenate3/4
  Matrix Concatenate/1 -> Matrix Concatenate7/1
  Matrix Concatenate1/1 -> Matrix Concatenate7/2
  Matrix Concatenate2/1 -> Matrix Concatenate7/3
  Matrix Concatenate3/1 -> Matrix Concatenate7/4
  Matrix Concatenate4/1 -> Matrix Concatenate7/5
  Matrix Concatenate7/1 -> M/1

== system mobilerobot_DT_SMC/tau/f2/S ==
  "fai " : Inport
  Constant19 : Constant  Value=c
  Constant20 : Constant  Value=-c
  Constant21 : Constant
  Constant22 : Constant  Value=0
  Constant23 : Constant  Value=0
  Constant24 : Constant
  Matrix Concatenate{1,3..6} (5 alike) : Concatenate  Mode=Multidimensional array  ConcatenateDimension=2
  Matrix Concatenate{7..9,11} (4 alike) : Concatenate  Mode=Multidimensional array
  Subsystem : Subsystem
  Subsystem1 : Subsystem
  Subsystem2 : Subsystem
  Subsystem3 : Subsystem
  S : Outport
  wires:
  Constant19/1 -> Matrix Concatenate4/1
  Constant23/1 -> Matrix Concatenate5/2
  Constant21/1 -> Matrix Concatenate5/1
  Matrix Concatenate6/1 -> Matrix Concatenate11/2
  Subsystem3/1(Out1) -> Matrix Concatenate1/1
  Subsystem2/1(Out1) -> Matrix Concatenate1/2
  Matrix Concatenate9/1 -> Matrix Concatenate11/1
  Subsystem1/1(Out1) -> Matrix Concatenate3/1
  Matrix Concatenate4/1 -> Matrix Concatenate8/1
  Constant24/1 -> Matrix Concatenate6/2
  Matrix Concatenate5/1 -> Matrix Concatenate8/2
  Matrix Concatenate7/1 -> Matrix Concatenate9/1
  Subsystem/1(Out1) -> Matrix Concatenate3/2
  Constant20/1 -> Matrix Concatenate4/2
  Matrix Concatenate1/1 -> Matrix Concatenate7/1
  Matrix Concatenate3/1 -> Matrix Concatenate7/2
  Matrix Concatenate8/1 -> Matrix Concatenate9/2
  Matrix Concatenate11/1 -> S/1
  Constant22/1 -> Matrix Concatenate6/1
  "fai "/1 -> Subsystem/1("fai "), Subsystem1/1("fai "), Subsystem2/1("fai "), Subsystem3/1("fai ")

== system mobilerobot_DT_SMC/tau/f2/S1 ==
  "fai " : Inport
  Constant19 : Constant  Value=c
  Constant20 : Constant  Value=-c
  Constant21 : Constant
  Constant22 : Constant  Value=0
  Constant23 : Constant  Value=0
  Constant24 : Constant
  Matrix Concatenate{1,3..6} (5 alike) : Concatenate  Mode=Multidimensional array  ConcatenateDimension=2
  Matrix Concatenate{7..9,11} (4 alike) : Concatenate  Mode=Multidimensional array
  Subsystem : Subsystem
  Subsystem1 : Subsystem
  Subsystem2 : Subsystem
  Subsystem3 : Subsystem
  S : Outport
  wires:
  Constant19/1 -> Matrix Concatenate4/1
  Constant23/1 -> Matrix Concatenate5/2
  Constant21/1 -> Matrix Concatenate5/1
  Matrix Concatenate6/1 -> Matrix Concatenate11/2
  Subsystem3/1(Out1) -> Matrix Concatenate1/1
  Subsystem2/1(Out1) -> Matrix Concatenate1/2
  Matrix Concatenate9/1 -> Matrix Concatenate11/1
  Subsystem1/1(Out1) -> Matrix Concatenate3/1
  Matrix Concatenate4/1 -> Matrix Concatenate8/1
  Constant24/1 -> Matrix Concatenate6/2
  Matrix Concatenate5/1 -> Matrix Concatenate8/2
  Matrix Concatenate7/1 -> Matrix Concatenate9/1
  Subsystem/1(Out1) -> Matrix Concatenate3/2
  Constant20/1 -> Matrix Concatenate4/2
  Matrix Concatenate1/1 -> Matrix Concatenate7/1
  Matrix Concatenate3/1 -> Matrix Concatenate7/2
  Matrix Concatenate8/1 -> Matrix Concatenate9/2
  Matrix Concatenate11/1 -> S/1
  Constant22/1 -> Matrix Concatenate6/1
  "fai "/1 -> Subsystem/1("fai "), Subsystem1/1("fai "), Subsystem2/1("fai "), Subsystem3/1("fai ")

== system mobilerobot_DT_SMC/tau/f2/S_transpose  ==
  "fai " : Inport
  Constant19 : Constant  Value=c
  Constant20 : Constant  Value=-c
  Constant21 : Constant
  Constant22 : Constant  Value=0
  Constant23 : Constant  Value=0
  Constant24 : Constant
  Matrix Concatenate{1,3..6} (5 alike) : Concatenate  Mode=Multidimensional array
  Matrix Concatenate{7..9,11} (4 alike) : Concatenate  Mode=Multidimensional array  ConcatenateDimension=2
  Subsystem : Subsystem
  Subsystem1 : Subsystem
  Subsystem2 : Subsystem
  Subsystem3 : Subsystem
  S_t : Outport
  wires:
  Subsystem/1(Out1) -> Matrix Concatenate3/2
  Constant20/1 -> Matrix Concatenate4/2
  Matrix Concatenate1/1 -> Matrix Concatenate7/1
  Subsystem3/1(Out1) -> Matrix Concatenate1/1
  "fai "/1 -> Subsystem/1("fai "), Subsystem1/1("fai "), Subsystem2/1("fai "), Subsystem3/1("fai ")
  Matrix Concatenate3/1 -> Matrix Concatenate7/2
  Constant19/1 -> Matrix Concatenate4/1
  Matrix Concatenate7/1 -> Matrix Concatenate9/1
  Constant24/1 -> Matrix Concatenate6/2
  Constant22/1 -> Matrix Concatenate6/1
  Matrix Concatenate9/1 -> Matrix Concatenate11/1
  Matrix Concatenate5/1 -> Matrix Concatenate8/2
  Constant21/1 -> Matrix Concatenate5/1
  Matrix Concatenate6/1 -> Matrix Concatenate11/2
  Subsystem1/1(Out1) -> Matrix Concatenate3/1
  Matrix Concatenate8/1 -> Matrix Concatenate9/2
  Subsystem2/1(Out1) -> Matrix Concatenate1/2
  Matrix Concatenate4/1 -> Matrix Concatenate8/1
  Matrix Concatenate11/1 -> S_t/1
  Constant23/1 -> Matrix Concatenate5/2

== system mobilerobot_DT_SMC/tau/f2/S_transpose 1 ==
  "fai " : Inport
  Constant19 : Constant  Value=c
  Constant20 : Constant  Value=-c
  Constant21 : Constant
  Constant22 : Constant  Value=0
  Constant23 : Constant  Value=0
  Constant24 : Constant
  Matrix Concatenate{1,3..6} (5 alike) : Concatenate  Mode=Multidimensional array
  Matrix Concatenate{7..9,11} (4 alike) : Concatenate  Mode=Multidimensional array  ConcatenateDimension=2
  Subsystem : Subsystem
  Subsystem1 : Subsystem
  Subsystem2 : Subsystem
  Subsystem3 : Subsystem
  S_t : Outport
  wires:
  Subsystem/1(Out1) -> Matrix Concatenate3/2
  Constant20/1 -> Matrix Concatenate4/2
  Matrix Concatenate1/1 -> Matrix Concatenate7/1
  Subsystem3/1(Out1) -> Matrix Concatenate1/1
  "fai "/1 -> Subsystem/1("fai "), Subsystem1/1("fai "), Subsystem2/1("fai "), Subsystem3/1("fai ")
  Matrix Concatenate3/1 -> Matrix Concatenate7/2
  Constant19/1 -> Matrix Concatenate4/1
  Matrix Concatenate7/1 -> Matrix Concatenate9/1
  Constant24/1 -> Matrix Concatenate6/2
  Constant22/1 -> Matrix Concatenate6/1
  Matrix Concatenate9/1 -> Matrix Concatenate11/1
  Matrix Concatenate5/1 -> Matrix Concatenate8/2
  Constant21/1 -> Matrix Concatenate5/1
  Matrix Concatenate6/1 -> Matrix Concatenate11/2
  Subsystem1/1(Out1) -> Matrix Concatenate3/1
  Matrix Concatenate8/1 -> Matrix Concatenate9/2
  Subsystem2/1(Out1) -> Matrix Concatenate1/2
  Matrix Concatenate4/1 -> Matrix Concatenate8/1
  Matrix Concatenate11/1 -> S_t/1
  Constant23/1 -> Matrix Concatenate5/2

== system mobilerobot_DT_SMC/tau/f2/S_transpose 2 ==
  "fai " : Inport
  Constant19 : Constant  Value=c
  Constant20 : Constant  Value=-c
  Constant21 : Constant
  Constant22 : Constant  Value=0
  Constant23 : Constant  Value=0
  Constant24 : Constant
  Matrix Concatenate{1,3..6} (5 alike) : Concatenate  Mode=Multidimensional array
  Matrix Concatenate{7..9,11} (4 alike) : Concatenate  Mode=Multidimensional array  ConcatenateDimension=2
  Subsystem : Subsystem
  Subsystem1 : Subsystem
  Subsystem2 : Subsystem
  Subsystem3 : Subsystem
  S_t : Outport
  wires:
  Subsystem/1(Out1) -> Matrix Concatenate3/2
  Constant20/1 -> Matrix Concatenate4/2
  Matrix Concatenate1/1 -> Matrix Concatenate7/1
  Subsystem3/1(Out1) -> Matrix Concatenate1/1
  "fai "/1 -> Subsystem/1("fai "), Subsystem1/1("fai "), Subsystem2/1("fai "), Subsystem3/1("fai ")
  Matrix Concatenate3/1 -> Matrix Concatenate7/2
  Constant19/1 -> Matrix Concatenate4/1
  Matrix Concatenate7/1 -> Matrix Concatenate9/1
  Constant24/1 -> Matrix Concatenate6/2
  Constant22/1 -> Matrix Concatenate6/1
  Matrix Concatenate9/1 -> Matrix Concatenate11/1
  Matrix Concatenate5/1 -> Matrix Concatenate8/2
  Constant21/1 -> Matrix Concatenate5/1
  Matrix Concatenate6/1 -> Matrix Concatenate11/2
  Subsystem1/1(Out1) -> Matrix Concatenate3/1
  Matrix Concatenate8/1 -> Matrix Concatenate9/2
  Subsystem2/1(Out1) -> Matrix Concatenate1/2
  Matrix Concatenate4/1 -> Matrix Concatenate8/1
  Matrix Concatenate11/1 -> S_t/1
  Constant23/1 -> Matrix Concatenate5/2

== system mobilerobot_DT_SMC/tau/f2/V ==
  fai : Inport
  (fai_dot)^2 : Inport  Port=2
  Constant : Constant  Value=-m_c
  Constant1 : Constant  Value=-m_c
  Constant2 : Constant  Value=d
  Constant3 : Constant  Value=0
  Constant4 : Constant  Value=d
  Matrix Concatenate : Concatenate  NumInputs=5  Mode=Multidimensional array
  Product{,1..5} (6 alike) : Product
  Trigonometric Function : Trigonometry  Operator=cos
  Trigonometric Function1 : Trigonometry
  V : Outport
  wires:
  Constant1/1 -> Product3/1
  Constant2/1 -> Product3/2
  Product3/1 -> Product4/1
  Product4/1 -> Product5/1
  Trigonometric Function1/1 -> Product5/2
  (fai_dot)^2/1 -> Product4/2, Product1/2
  fai/1 -> Trigonometric Function1/1, Trigonometric Function/1
  Product1/1 -> Product2/1
  Constant4/1 -> Product/2
  Constant/1 -> Product/1
  Product/1 -> Product1/1
  Trigonometric Function/1 -> Product2/2
  Product2/1 -> Matrix Concatenate/1
  Product5/1 -> Matrix Concatenate/2
  Constant3/1 -> Matrix Concatenate/5, Matrix Concatenate/4, Matrix Concatenate/3
  Matrix Concatenate/1 -> V/1

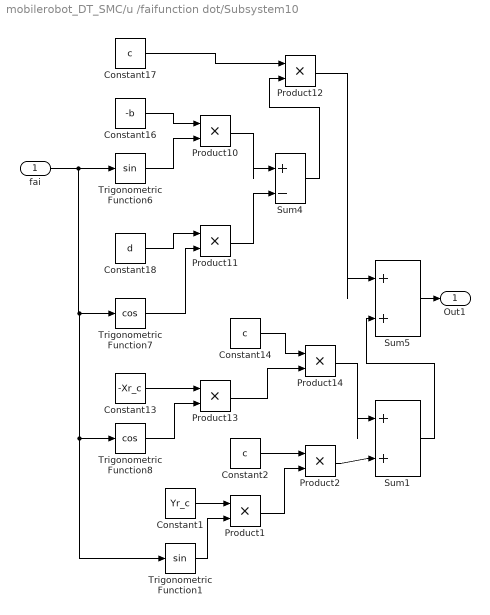
== system mobilerobot_DT_SMC/u /faifunction dot/Subsystem10 ==
  fai : Inport
  Constant1 : Constant  Value=Yr_c
  Constant13 : Constant  Value=-Xr_c
  Constant14 : Constant  Value=c
  Constant16 : Constant  Value=-b
  Constant17 : Constant  Value=c
  Constant18 : Constant  Value=d
  Constant2 : Constant  Value=c
  Product{1..2,10..14} (7 alike) : Product
  Sum1 : Sum  Inputs=|++
  Sum4 : Sum  Inputs=|+-
  Sum5 : Sum  Inputs=|++
  Trigonometric Function1 : Trigonometry
  Trigonometric Function6 : Trigonometry
  Trigonometric Function7 : Trigonometry  Operator=cos
  Trigonometric Function8 : Trigonometry  Operator=cos
  Out1 : Outport
  wires:
  Constant16/1 -> Product10/1
  Constant14/1 -> Product14/1
  Constant13/1 -> Product13/1
  Trigonometric Function6/1 -> Product10/2
  Trigonometric Function7/1 -> Product11/2
  Product13/1 -> Product14/2
  Product12/1 -> Sum5/1
  Sum4/1 -> Product12/2
  Constant17/1 -> Product12/1
  fai/1 -> Trigonometric Function1/1, Trigonometric Function8/1, Trigonometric Function7/1, Trigonometric Function6/1
  Constant18/1 -> Product11/1
  Trigonometric Function8/1 -> Product13/2
  Product11/1 -> Sum4/2
  Product10/1 -> Sum4/1
  Sum5/1 -> Out1/1
  Constant1/1 -> Product1/1
  Trigonometric Function1/1 -> Product1/2
  Constant2/1 -> Product2/1
  Product1/1 -> Product2/2
  Product14/1 -> Sum1/1
  Product2/1 -> Sum1/2
  Sum1/1 -> Sum5/2

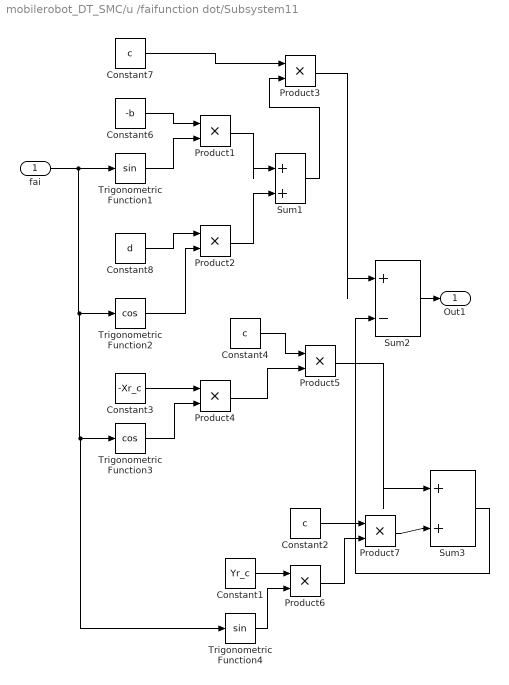
== system mobilerobot_DT_SMC/u /faifunction dot/Subsystem11 ==
  fai : Inport
  Constant1 : Constant  Value=Yr_c
  Constant2 : Constant  Value=c
  Constant3 : Constant  Value=-Xr_c
  Constant4 : Constant  Value=c
  Constant6 : Constant  Value=-b
  Constant7 : Constant  Value=c
  Constant8 : Constant  Value=d
  Product{1..7} (7 alike) : Product
  Sum1 : Sum  Inputs=|++
  Sum2 : Sum  Inputs=|+-
  Sum3 : Sum  Inputs=|++
  Trigonometric Function1 : Trigonometry
  Trigonometric Function2 : Trigonometry  Operator=cos
  Trigonometric Function3 : Trigonometry  Operator=cos
  Trigonometric Function4 : Trigonometry
  Out1 : Outport
  wires:
  Trigonometric Function2/1 -> Product2/2
  fai/1 -> Trigonometric Function4/1, Trigonometric Function3/1, Trigonometric Function2/1, Trigonometric Function1/1
  Sum1/1 -> Product3/2
  Constant8/1 -> Product2/1
  Constant3/1 -> Product4/1
  Product2/1 -> Sum1/2
  Constant4/1 -> Product5/1
  Product4/1 -> Product5/2
  Trigonometric Function1/1 -> Product1/2
  Product1/1 -> Sum1/1
  Product3/1 -> Sum2/1
  Constant7/1 -> Product3/1
  Trigonometric Function3/1 -> Product4/2
  Constant6/1 -> Product1/1
  Sum2/1 -> Out1/1
  Constant1/1 -> Product6/1
  Trigonometric Function4/1 -> Product6/2
  Product6/1 -> Product7/2
  Product7/1 -> Sum3/2
  Product5/1 -> Sum3/1
  Sum3/1 -> Sum2/2
  Constant2/1 -> Product7/1

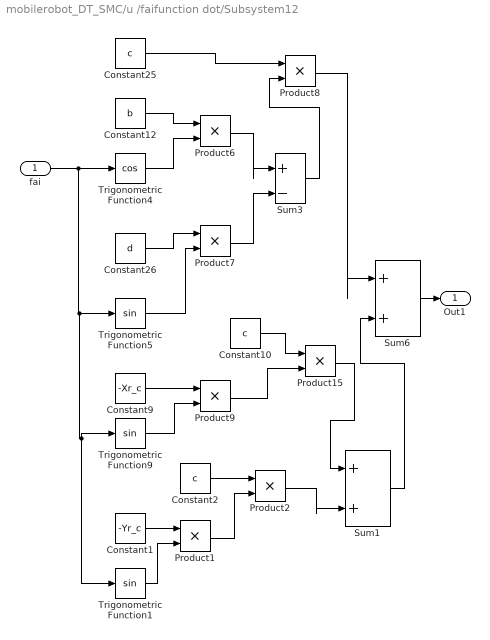
== system mobilerobot_DT_SMC/u /faifunction dot/Subsystem12 ==
  fai : Inport
  Constant1 : Constant  Value=-Yr_c
  Constant10 : Constant  Value=c
  Constant12 : Constant  Value=b
  Constant2 : Constant  Value=c
  Constant25 : Constant  Value=c
  Constant26 : Constant  Value=d
  Constant9 : Constant  Value=-Xr_c
  Product{1..2,6..9,15} (7 alike) : Product
  Sum1 : Sum  Inputs=|++
  Sum3 : Sum  Inputs=|+-
  Sum6 : Sum  Inputs=|++
  Trigonometric Function1 : Trigonometry
  Trigonometric Function4 : Trigonometry  Operator=cos
  Trigonometric Function5 : Trigonometry
  Trigonometric Function9 : Trigonometry
  Out1 : Outport
  wires:
  Sum6/1 -> Out1/1
  Sum3/1 -> Product8/2
  Trigonometric Function4/1 -> Product6/2
  Product6/1 -> Sum3/1
  Constant12/1 -> Product6/1
  Constant10/1 -> Product15/1
  Trigonometric Function5/1 -> Product7/2
  Product8/1 -> Sum6/1
  Product7/1 -> Sum3/2
  Trigonometric Function9/1 -> Product9/2
  Constant26/1 -> Product7/1
  Constant9/1 -> Product9/1
  Product9/1 -> Product15/2
  fai/1 -> Trigonometric Function1/1, Trigonometric Function9/1, Trigonometric Function5/1, Trigonometric Function4/1
  Constant25/1 -> Product8/1
  Constant1/1 -> Product1/1
  Trigonometric Function1/1 -> Product1/2
  Product1/1 -> Product2/2
  Constant2/1 -> Product2/1
  Product2/1 -> Sum1/2
  Product15/1 -> Sum1/1
  Sum1/1 -> Sum6/2

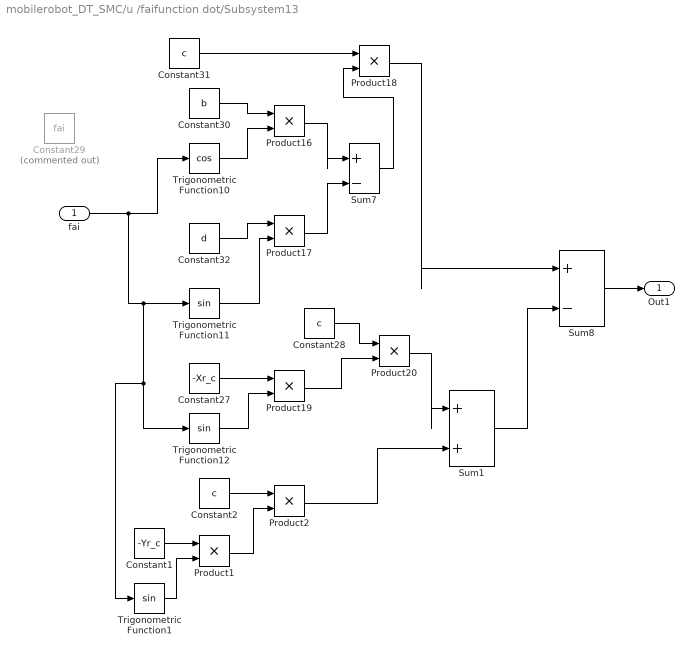
== system mobilerobot_DT_SMC/u /faifunction dot/Subsystem13 ==
  fai : Inport
  Constant1 : Constant  Value=-Yr_c
  Constant2 : Constant  Value=c
  Constant27 : Constant  Value=-Xr_c
  Constant28 : Constant  Value=c
  Constant29 : Constant  Commented=on  Value=fai
  Constant30 : Constant  Value=b
  Constant31 : Constant  Value=c
  Constant32 : Constant  Value=d
  Product{1..2,16..20} (7 alike) : Product
  Sum1 : Sum  Inputs=|++
  Sum7 : Sum  Inputs=|+-
  Sum8 : Sum  Inputs=|+-
  Trigonometric Function1 : Trigonometry
  Trigonometric Function10 : Trigonometry  Operator=cos
  Trigonometric Function11 : Trigonometry
  Trigonometric Function12 : Trigonometry
  Out1 : Outport
  wires:
  Product16/1 -> Sum7/1
  Constant28/1 -> Product20/1
  Constant27/1 -> Product19/1
  Constant32/1 -> Product17/1
  Product18/1 -> Sum8/1
  Trigonometric Function12/1 -> Product19/2
  Constant30/1 -> Product16/1
  Product17/1 -> Sum7/2
  Sum7/1 -> Product18/2
  Constant31/1 -> Product18/1
  Trigonometric Function10/1 -> Product16/2
  Trigonometric Function11/1 -> Product17/2
  Sum8/1 -> Out1/1
  Product19/1 -> Product20/2
  fai/1 -> Trigonometric Function1/1, Trigonometric Function12/1, Trigonometric Function11/1, Trigonometric Function10/1
  Constant1/1 -> Product1/1
  Trigonometric Function1/1 -> Product1/2
  Product1/1 -> Product2/2
  Constant2/1 -> Product2/1
  Product20/1 -> Sum1/1
  Product2/1 -> Sum1/2
  Sum1/1 -> Sum8/2

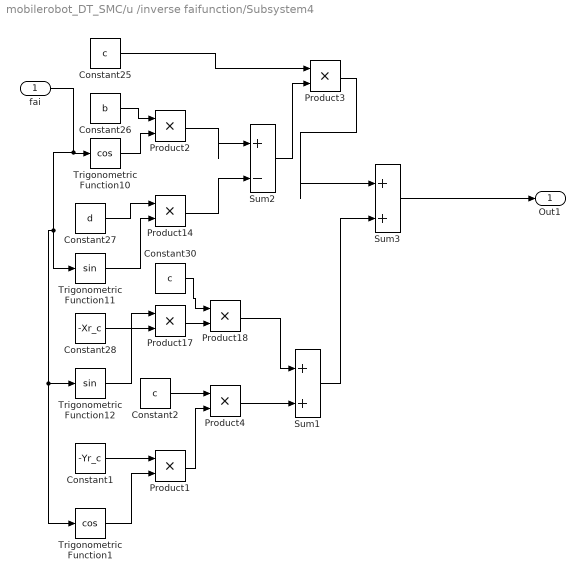
== system mobilerobot_DT_SMC/u /inverse faifunction/Subsystem4 ==
  "fai " : Inport
  Constant1 : Constant  Value=-Yr_c
  Constant2 : Constant  Value=c
  Constant25 : Constant  Value=c
  Constant26 : Constant  Value=b
  Constant27 : Constant  Value=d
  Constant28 : Constant  Value=-Xr_c
  Constant30 : Constant  Value=c
  Product{1..4,14,17..18} (7 alike) : Product
  Sum1 : Sum  Inputs=|++
  Sum2 : Sum  Inputs=|+-
  Sum3 : Sum  Inputs=|++
  Trigonometric Function1 : Trigonometry  Operator=cos
  Trigonometric Function10 : Trigonometry  Operator=cos
  Trigonometric Function11 : Trigonometry
  Trigonometric Function12 : Trigonometry
  Out1 : Outport
  wires:
  Trigonometric Function10/1 -> Product2/2
  Constant26/1 -> Product2/1
  Product14/1 -> Sum2/2
  Sum2/1 -> Product3/2
  Sum3/1 -> Out1/1
  Trigonometric Function12/1 -> Product17/1
  "fai "/1 -> Trigonometric Function1/1, Trigonometric Function12/1, Trigonometric Function11/1, Trigonometric Function10/1
  Constant27/1 -> Product14/1
  Product17/1 -> Product18/2
  Constant28/1 -> Product17/2
  Trigonometric Function11/1 -> Product14/2
  Constant30/1 -> Product18/1
  Product2/1 -> Sum2/1
  Product3/1 -> Sum3/1
  Constant25/1 -> Product3/1
  Constant1/1 -> Product1/1
  Trigonometric Function1/1 -> Product1/2
  Constant2/1 -> Product4/1
  Product1/1 -> Product4/2
  Product4/1 -> Sum1/2
  Product18/1 -> Sum1/1
  Sum1/1 -> Sum3/2
